simulink model "fig10_53and54a"  (Simulink 7.0)
settings: Solver=ode23  SolverMode=SingleTasking  StartTime=0.0  StopTime=20.0  RelTol=1e-3  AbsTol=1e-5
settings Model: Creator=abbas  LastModifiedBy=abbas  ExtModeTrigMode=oneshot  ExtModeArmWhenConnect=off
settings DataIOCC: LimitDataPoints=off
settings OptimizationCC: BlockReduction=off  BooleanDataType=off  InlineInvariantSignals=on
settings DebuggingCC: SaveWithParameterizedLinksMsg=none  SignalResolutionControl=TryResolveAllWithWarning  SolverPrmCheckMsg=none  MultiTaskDSMMsg=warning  MultiTaskCondExecSysMsg=none  StrictBusMsg=None
settings HardwareCC: TargetUnknown=on
settings RTWCC: IncludeERTFirstTime=on
settings GRTTargetCC: TargetFcnLib=ansi_tfl_tmw.mat  ModelReferenceCompliant=off  MatFileLogging=off

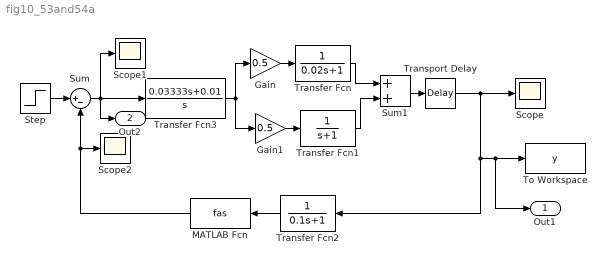
== system fig10_53and54a ==
  Gain : Gain  Gain=0.5  ParameterDataType=sfix(16)  ParameterScaling=2^0  OutDataType=sfix(16)  OutScaling=2^0  SaturateOnIntegerOverflow=on
  Gain1 : Gain  Gain=0.5  ParameterDataType=sfix(16)  ParameterScaling=2^0  OutDataType=sfix(16)  OutScaling=2^0  SaturateOnIntegerOverflow=on
  MATLAB Fcn : MATLABFcn  Orientation=left  MATLABFcn=fas  OutputDimensions=1
  Scope : Scope
      settings: TickLabels=on  DataFormat=Array
  Scope1 : Scope
      settings: TickLabels=on  DataFormat=Array
  Scope2 : Scope
      settings: TickLabels=on  DataFormat=Array
  Step : Step  Time=0  After=0.5
  Sum : Sum  Inputs=|+-  OutDataType=sfix(16)  OutScaling=2^0  SaturateOnIntegerOverflow=on  InputSameDT=on
  Sum1 : Sum  OutDataType=sfix(16)  OutScaling=2^0  SaturateOnIntegerOverflow=on  InputSameDT=on
  To Workspace : ToWorkspace  VariableName=y  SampleTime=-1  SaveFormat=Array
  Transfer Fcn : TransferFcn  Denominator=[0.02 1]
  Transfer Fcn1 : TransferFcn  Denominator=[1 1]
  Transfer Fcn2 : TransferFcn  Orientation=left  Denominator=[0.1 1]
  Transfer Fcn3 : TransferFcn  Numerator=[0.03333 0.01]  Denominator=[1 0]
  Transport Delay : TransportDelay  DelayTime=0.2
  Out1 : Outport  OutDataType=sfix(16)  OutScaling=2^0
  Out2 : Outport  Port=2  OutDataType=sfix(16)  OutScaling=2^0
  wires:
  Transfer Fcn1/1 -> Sum1/2
  Sum1/1 -> Transport Delay/1
  Transport Delay/1 -> Scope/1, Transfer Fcn2/1, To Workspace/1, Out1/1
  Transfer Fcn/1 -> Sum1/1
  Gain/1 -> Transfer Fcn/1
  Transfer Fcn3/1 -> Gain/1, Gain1/1
  Gain1/1 -> Transfer Fcn1/1
  Transfer Fcn2/1 -> MATLAB Fcn/1
  MATLAB Fcn/1 -> Scope2/1, Sum/2
  Step/1 -> Sum/1
  Sum/1 -> Transfer Fcn3/1, Scope1/1, Out2/1
